simulink model "quadcopter_control"  (R2018b)
settings: Solver=VariableStepAuto  StartTime=0.0  StopTime=2.5  RelTol=1e-3
undefined symbols (not defined in the file or in its folder): armLength, dragFactor, iX, iY, iZ, mass, phi0, phiDot0, psi0, psiDot0, theta0, thetaDot0, thrustFactor, trajectory, Ts, x0, xDot0, y0, yDot0, z0, zDot0
libraries: simulink x1
settings Model: Creator=Ramprasad  LastModifiedBy=Ramprasad

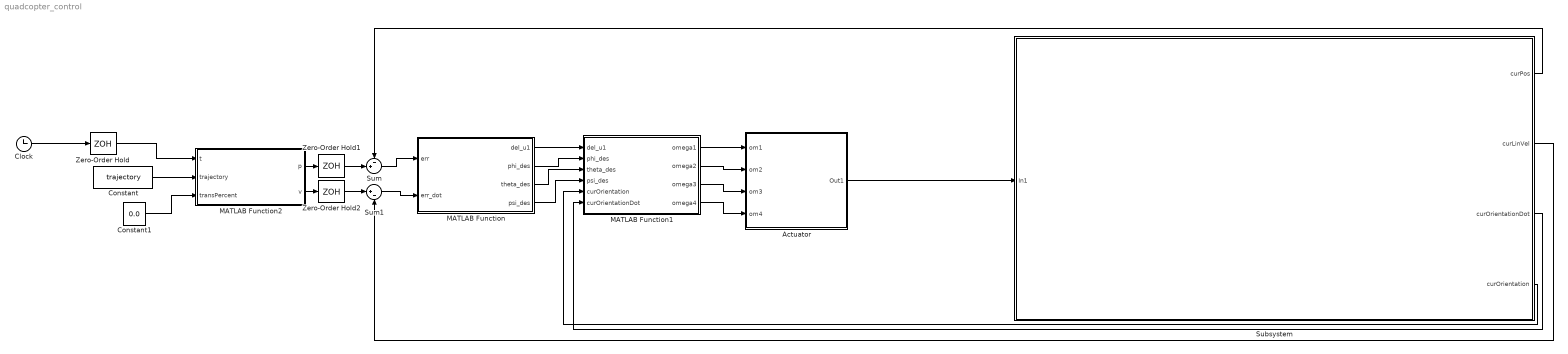
== system quadcopter_control ==
  Actuator : Subsystem
  Clock : Clock
  Constant : Constant  Value=trajectory
  Constant1 : Constant  Value=0.0
  MATLAB Function : MATLAB Function  TreatAsAtomicUnit=on
  MATLAB Function1 : MATLAB Function  TreatAsAtomicUnit=on
  MATLAB Function2 : MATLAB Function  TreatAsAtomicUnit=on
  Subsystem : Subsystem
  Sum : Sum  Inputs=-+|
  Sum1 : Sum  Inputs=|+-
  Zero-Order Hold : ZeroOrderHold  SampleTime=0.001
  Zero-Order Hold1 : ZeroOrderHold  SampleTime=0.001
  Zero-Order Hold2 : ZeroOrderHold  SampleTime=0.001
  wires:
  Actuator/1(Out1) -> Subsystem/1(In1)
  Constant/1 -> MATLAB Function2/2(trajectory)
  Clock/1 -> Zero-Order Hold/1
  Zero-Order Hold/1 -> MATLAB Function2/1(t)
  Subsystem/3(curOrientationDot) -> MATLAB Function1/6(curOrientationDot)
  Subsystem/4(curOrientation) -> MATLAB Function1/5(curOrientation)
  MATLAB Function/1(del_u1) -> MATLAB Function1/1(del_u1)
  MATLAB Function/2(phi_des) -> MATLAB Function1/2(phi_des)
  MATLAB Function/3(theta_des) -> MATLAB Function1/3(theta_des)
  MATLAB Function/4(psi_des) -> MATLAB Function1/4(psi_des)
  MATLAB Function2/1(p) -> Zero-Order Hold1/1
  MATLAB Function2/2(v) -> Zero-Order Hold2/1
  Zero-Order Hold1/1 -> Sum/2
  Zero-Order Hold2/1 -> Sum1/1
  Sum/1 -> MATLAB Function/1(err)
  Sum1/1 -> MATLAB Function/2(err_dot)
  MATLAB Function1/1(omega1) -> Actuator/1(om1)
  MATLAB Function1/2(omega2) -> Actuator/2(om2)
  MATLAB Function1/3(omega3) -> Actuator/3(om3)
  MATLAB Function1/4(omega4) -> Actuator/4(om4)
  Subsystem/2(curLinVel) -> Sum1/2
  Subsystem/1(curPos) -> Sum/1
  Constant1/1 -> MATLAB Function2/3(transPercent)

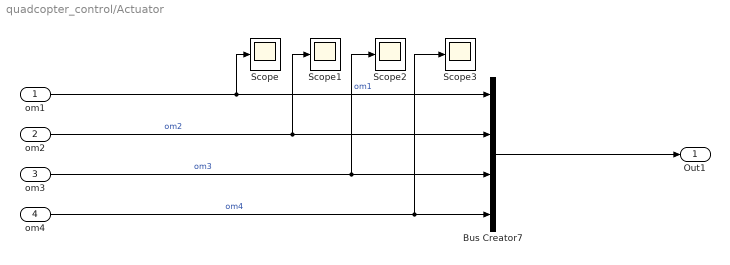
== system quadcopter_control/Actuator ==
  om1 : Inport
  om2 : Inport  Port=2
  om3 : Inport  Port=3
  om4 : Inport  Port=4
  Bus Creator7 : BusCreator  Inputs=4
  Scope{,1..3} (4 alike) : Scope
  Out1 : Outport
  wires:
  om1/1 -> Scope/1, Bus Creator7/1  "om1"
  om4/1 -> Scope3/1, Bus Creator7/4  "om4"
  Bus Creator7/1 -> Out1/1
  om2/1 -> Scope1/1, Bus Creator7/2  "om2"
  om3/1 -> Scope2/1, Bus Creator7/3  "om3"

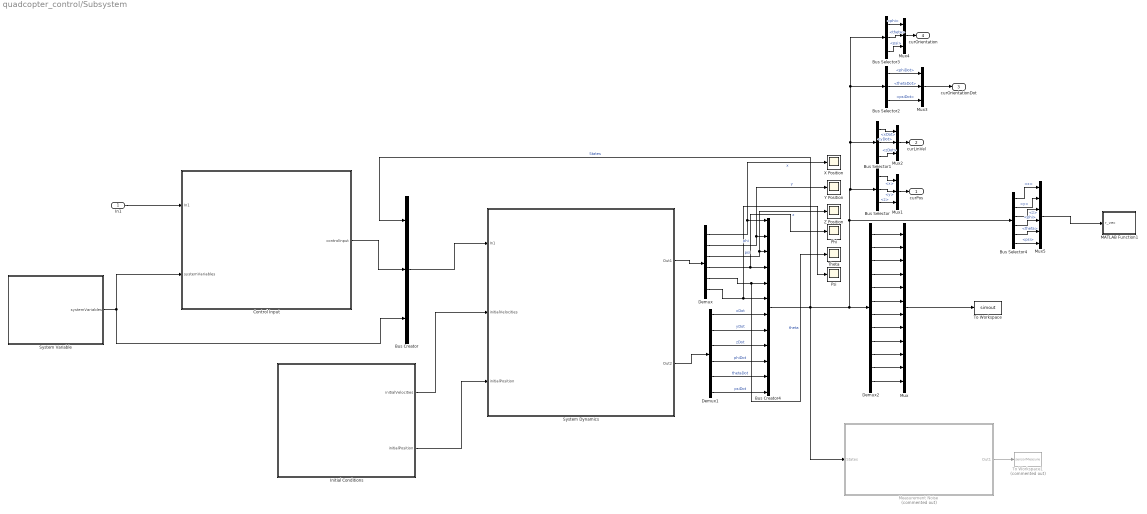
== system quadcopter_control/Subsystem ==
  In1 : Inport
  Bus Creator : BusCreator  Inputs=3
  Bus Creator4 : BusCreator  Inputs=12
  Bus Selector : BusSelector  OutputSignals=x,y,z
  Bus Selector1 : BusSelector  OutputSignals=xDot,yDot,zDot
  Bus Selector2 : BusSelector  OutputSignals=phiDot,thetaDot,psiDot
  Bus Selector3 : BusSelector  OutputSignals=phi,theta,psi
  Bus Selector4 : BusSelector  OutputSignals=x,y,z,phi,theta,psi
  Control Input : Subsystem
  Demux : Demux  Outputs=6
  Demux1 : Demux  Outputs=6
  Demux2 : Demux  Outputs=12
  Initial Conditions : Subsystem
  MATLAB Function1 : MATLAB Function  TreatAsAtomicUnit=on
  Measurement Noise : Subsystem  Commented=on
  Mux : Mux  Inputs=12
  Mux{1..4} (4 alike) : Mux  Inputs=3
  Mux5 : Mux  Inputs=6
  Phi : Scope
  Psi : Scope
  System Dynamics : Subsystem
  System Variable : Subsystem
  Theta : Scope
  To Workspace : ToWorkspace  VariableName=simout  SaveFormat=Timeseries  SampleTime=-1
  To Workspace1 : ToWorkspace  Commented=on  VariableName=sensorMeasure  SaveFormat=Timeseries  SampleTime=-1
  X Position : Scope
  Y Position : Scope
  Z Position : Scope
  curPos : Outport
  curLinVel : Outport  Port=2
  curOrientationDot : Outport  Port=3
  curOrientation : Outport  Port=4
  wires:
  Demux1/1 -> Bus Creator4/7  "xDot"
  Demux2/6 -> Mux/6
  Demux/6 -> Psi/1, Bus Creator4/6  "psi"
  Demux1/2 -> Bus Creator4/8  "yDot"
  Mux/1 -> To Workspace/1
  Demux2/9 -> Mux/9
  Demux1/6 -> Bus Creator4/12  "psiDot"
  Measurement Noise/1(Out1) -> To Workspace1/1
  Demux/4 -> Phi/1, Bus Creator4/4  "phi"
  System Dynamics/1(Out1) -> Demux/1
  Initial Conditions/1(initialVelocities) -> System Dynamics/2(initialVelocities)
  Initial Conditions/2(initialPosition) -> System Dynamics/3(initialPosition)
  Bus Creator/1 -> System Dynamics/1(In1)
  Demux/2 -> Bus Creator4/2, Y Position/1  "y"
  Demux2/5 -> Mux/5
  System Dynamics/2(Out2) -> Demux1/1
  Demux2/3 -> Mux/3
  Demux/1 -> Bus Creator4/1, X Position/1  "x"
  Demux2/8 -> Mux/8
  Demux2/7 -> Mux/7
  Control Input/1(controlInput) -> Bus Creator/2
  Demux2/2 -> Mux/2
  In1/1 -> Control Input/1(In1)
  Demux2/12 -> Mux/12
  Demux1/4 -> Bus Creator4/10  "phiDot"
  Demux/5 -> Theta/1, Bus Creator4/5  "theta"
  Demux/3 -> Z Position/1, Bus Creator4/3  "z"
  Demux2/1 -> Mux/1
  Demux2/10 -> Mux/10
  Bus Creator4/1 -> Bus Creator/1, Bus Selector3/1, Bus Selector2/1, Bus Selector1/1, Bus Selector/1, Bus Selector4/1, Demux2/1, Measurement Noise/1(States)  "States"
  Demux2/11 -> Mux/11
  Demux1/5 -> Bus Creator4/11  "thetaDot"
  Demux2/4 -> Mux/4
  Demux1/3 -> Bus Creator4/9  "zDot"
  System Variable/1(systemVariables) -> Control Input/2(systemVariables), Bus Creator/3
  Bus Selector/3 -> Mux1/3  "<z>"
  Bus Selector/2 -> Mux1/2  "<y>"
  Bus Selector/1 -> Mux1/1  "<x>"
  Mux1/1 -> curPos/1
  Bus Selector1/2 -> Mux2/2  "<yDot>"
  Bus Selector1/3 -> Mux2/3  "<zDot>"
  Bus Selector1/1 -> Mux2/1  "<xDot>"
  Mux2/1 -> curLinVel/1
  Bus Selector3/1 -> Mux4/1  "<phi>"
  Bus Selector3/2 -> Mux4/2  "<theta>"
  Bus Selector3/3 -> Mux4/3  "<psi>"
  Mux4/1 -> curOrientation/1
  Bus Selector2/1 -> Mux3/1  "<phiDot>"
  Bus Selector2/2 -> Mux3/2  "<thetaDot>"
  Mux3/1 -> curOrientationDot/1
  Bus Selector2/3 -> Mux3/3  "<psiDot>"
  Bus Selector4/1 -> Mux5/1  "<x>"
  Bus Selector4/2 -> Mux5/2  "<y>"
  Bus Selector4/3 -> Mux5/3  "<z>"
  Bus Selector4/4 -> Mux5/4  "<phi>"
  Bus Selector4/5 -> Mux5/5  "<theta>"
  Bus Selector4/6 -> Mux5/6  "<psi>"
  Mux5/1 -> MATLAB Function1/1(r_vec)

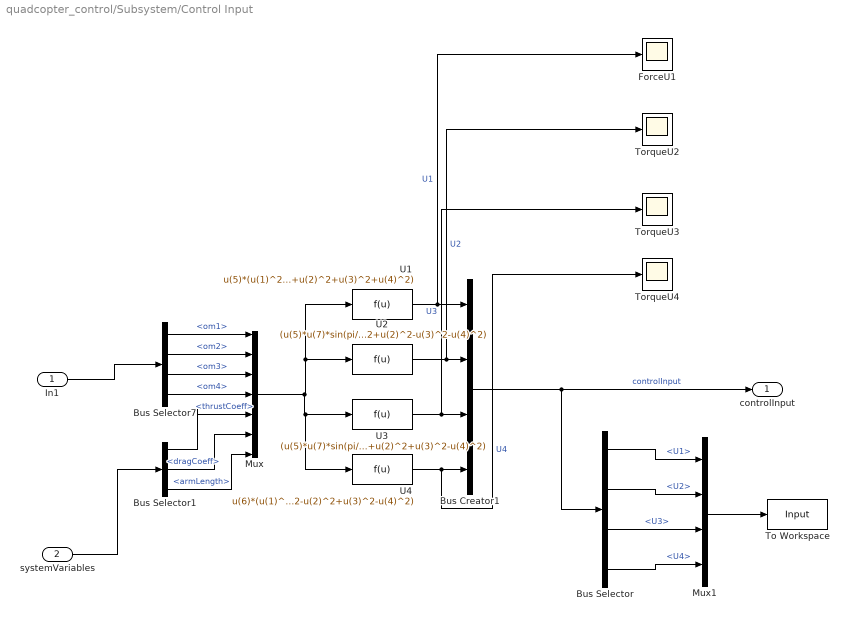
== system quadcopter_control/Subsystem/Control Input ==
  In1 : Inport
  systemVariables : Inport  Port=2
  Bus Creator1 : BusCreator  Inputs=4
  Bus Selector : BusSelector  OutputSignals=U1,U2,U3,U4
  Bus Selector1 : BusSelector  OutputSignals=thrustCoeff,dragCoeff,armLength
  Bus Selector7 : BusSelector  OutputSignals=om1,om2,om3,om4
  ForceU1 : Scope
  Mux : Mux  Inputs=7
  Mux1 : Mux
  To Workspace : ToWorkspace  VariableName=Input  SaveFormat=Timeseries  SampleTime=-1
  TorqueU2 : Scope
  TorqueU3 : Scope
  TorqueU4 : Scope
  U1 : Fcn  Expr=u(5)*(u(1)^2+u(2)^2+u(3)^2+u(4)^2)
  U2 : Fcn  Expr=(u(5)*u(7)*sin(pi/4))*(u(1)^2+u(2)^2-u(3)^2-u(4)^2)
  U3 : Fcn  Expr=(u(5)*u(7)*sin(pi/4))*(-u(1)^2+u(2)^2+u(3)^2-u(4)^2)
  U4 : Fcn  Expr=u(6)*(u(1)^2-u(2)^2+u(3)^2-u(4)^2)
  controlInput : Outport
  wires:
  Mux1/1 -> To Workspace/1
  Bus Selector/4 -> Mux1/4  "<U4>"
  Bus Selector/3 -> Mux1/3  "<U3>"
  Bus Selector/2 -> Mux1/2  "<U2>"
  Bus Selector/1 -> Mux1/1  "<U1>"
  Bus Selector7/3 -> Mux/3  "<om3>"
  In1/1 -> Bus Selector7/1
  Mux/1 -> U1/1, U2/1, U3/1, U4/1
  U1/1 -> Bus Creator1/1, ForceU1/1  "U1"
  U4/1 -> Bus Creator1/4, TorqueU4/1  "U4"
  Bus Selector1/3 -> Mux/7  "<armLength>"
  U3/1 -> Bus Creator1/3, TorqueU3/1  "U3"
  Bus Selector1/1 -> Mux/5  "<thrustCoeff>"
  Bus Creator1/1 -> controlInput/1, Bus Selector/1  "controlInput"
  Bus Selector1/2 -> Mux/6  "<dragCoeff>"
  U2/1 -> Bus Creator1/2, TorqueU2/1  "U2"
  Bus Selector7/1 -> Mux/1  "<om1>"
  Bus Selector7/4 -> Mux/4  "<om4>"
  Bus Selector7/2 -> Mux/2  "<om2>"
  systemVariables/1 -> Bus Selector1/1

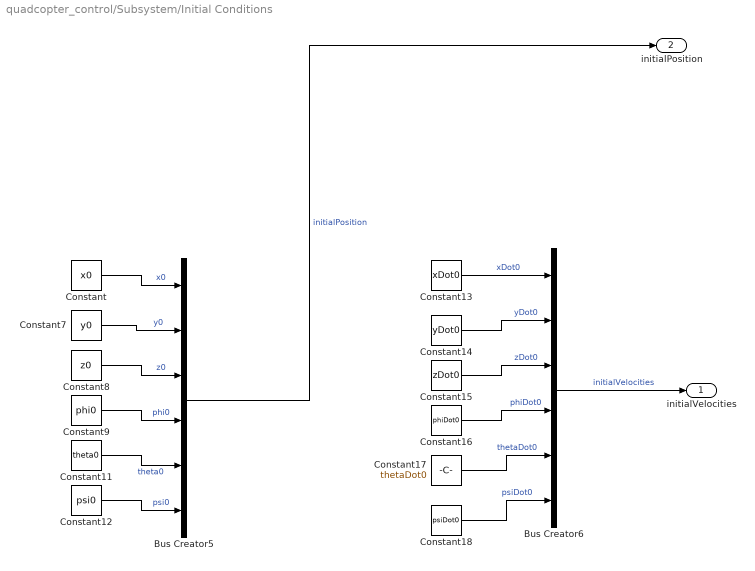
== system quadcopter_control/Subsystem/Initial Conditions ==
  Bus Creator5 : BusCreator  Inputs=6
  Bus Creator6 : BusCreator  Inputs=6
  Constant : Constant  Value=x0
  Constant11 : Constant  Value=theta0
  Constant12 : Constant  Value=psi0
  Constant13 : Constant  Value=xDot0
  Constant14 : Constant  Value=yDot0
  Constant15 : Constant  Value=zDot0
  Constant16 : Constant  Value=phiDot0
  Constant17 : Constant  Value=thetaDot0
  Constant18 : Constant  Value=psiDot0
  Constant7 : Constant  Value=y0
  Constant8 : Constant  Value=z0
  Constant9 : Constant  Value=phi0
  initialVelocities : Outport
  initialPosition : Outport  Port=2
  wires:
  Constant9/1 -> Bus Creator5/4  "phi0"
  Constant14/1 -> Bus Creator6/2  "yDot0"
  Constant17/1 -> Bus Creator6/5  "thetaDot0"
  Constant18/1 -> Bus Creator6/6  "psiDot0"
  Constant13/1 -> Bus Creator6/1  "xDot0"
  Constant11/1 -> Bus Creator5/5  "theta0"
  Constant8/1 -> Bus Creator5/3  "z0"
  Constant16/1 -> Bus Creator6/4  "phiDot0"
  Constant12/1 -> Bus Creator5/6  "psi0"
  Constant15/1 -> Bus Creator6/3  "zDot0"
  Constant/1 -> Bus Creator5/1  "x0"
  Bus Creator6/1 -> initialVelocities/1  "initialVelocities"
  Constant7/1 -> Bus Creator5/2  "y0"
  Bus Creator5/1 -> initialPosition/1  "initialPosition"

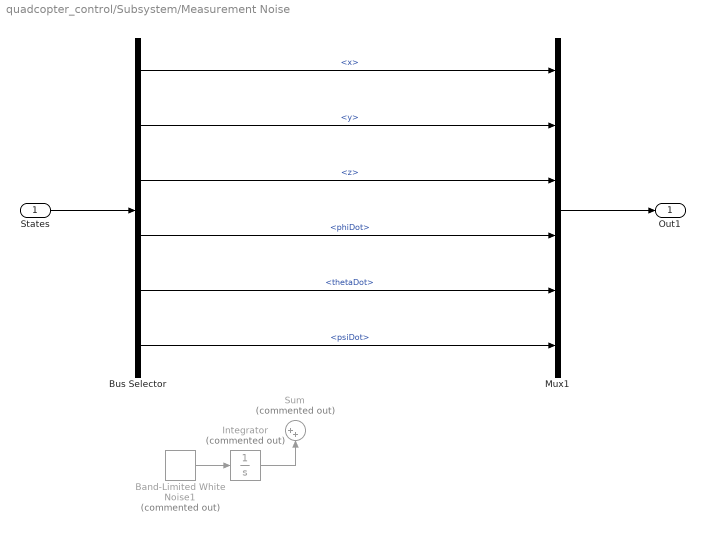
== system quadcopter_control/Subsystem/Measurement Noise ==
  States : Inport
  Band-Limited White Noise1 : simulink/Sources/Band-Limited White Noise  Commented=on  Cov=[0.0]  Ts=Ts  seed=[23341]
  Bus Selector : BusSelector  OutputSignals=x,y,z,phiDot,thetaDot,psiDot
  Integrator : Integrator  Commented=on
  Mux1 : Mux  Inputs=6
  Sum : Sum  Commented=on  Inputs=|++
  Out1 : Outport
  wires:
  Integrator/1 -> Sum/2
  Bus Selector/3 -> Mux1/3  "<z>"
  Bus Selector/2 -> Mux1/2  "<y>"
  Mux1/1 -> Out1/1
  Band-Limited White Noise1/1 -> Integrator/1
  Bus Selector/4 -> Mux1/4  "<phiDot>"
  States/1 -> Bus Selector/1
  Bus Selector/6 -> Mux1/6  "<psiDot>"
  Bus Selector/5 -> Mux1/5  "<thetaDot>"
  Bus Selector/1 -> Mux1/1  "<x>"

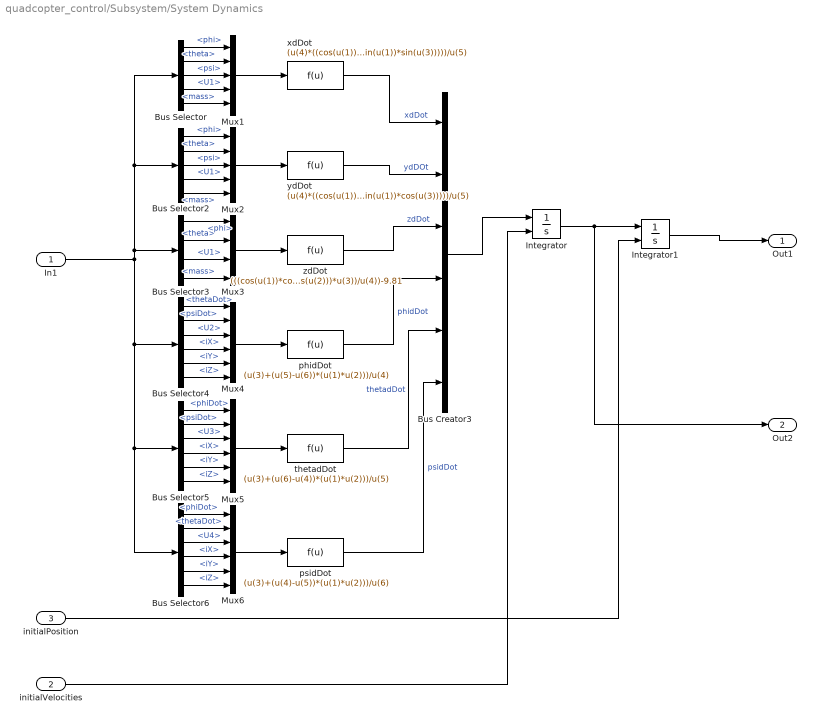
== system quadcopter_control/Subsystem/System Dynamics ==
  In1 : Inport
  initialVelocities : Inport  Port=2
  initialPosition : Inport  Port=3
  Bus Creator3 : BusCreator  Inputs=6
  Bus Selector : BusSelector  OutputSignals=States.phi,States.theta,States.psi,controlInput.U1,systemVariables.mass
  Bus Selector2 : BusSelector  OutputSignals=States.phi,States.theta,States.psi,controlInput.U1,systemVariables.mass
  Bus Selector3 : BusSelector  OutputSignals=States.phi,States.theta,controlInput.U1,systemVariables.mass
  Bus Selector4 : BusSelector  OutputSignals=States.thetaDot,States.psiDot,controlInput.U2,systemVariables.iX,systemVariables.iY,systemVariables.iZ
  Bus Selector5 : BusSelector  OutputSignals=States.phiDot,States.psiDot,controlInput.U3,systemVariables.iX,systemVariables.iY,systemVariables.iZ
  Bus Selector6 : BusSelector  OutputSignals=States.phiDot,States.thetaDot,controlInput.U4,systemVariables.iX,systemVariables.iY,systemVariables.iZ
  Integrator : Integrator  InitialConditionSource=external
  Integrator1 : Integrator  InitialConditionSource=external
  Mux1 : Mux  Inputs=5
  Mux2 : Mux  Inputs=5
  Mux3 : Mux
  Mux4 : Mux  Inputs=6
  Mux5 : Mux  Inputs=6
  Mux6 : Mux  Inputs=6
  phidDot : Fcn  Expr=(u(3)+(u(5)-u(6))*(u(1)*u(2)))/u(4)
  psidDot : Fcn  Expr=(u(3)+(u(4)-u(5))*(u(1)*u(2)))/u(6)
  thetadDot : Fcn  Expr=(u(3)+(u(6)-u(4))*(u(1)*u(2)))/u(5)
  xdDot : Fcn  Expr=(u(4)*((cos(u(1))*sin(u(2))*cos(u(3)))+(sin(u(1))*sin(u(3)))))/u(5)
  ydDot : Fcn  Expr=(u(4)*((cos(u(1))*sin(u(2))*sin(u(3)))-(sin(u(1))*cos(u(3)))))/u(5)
  zdDot : Fcn  Expr=(((cos(u(1))*cos(u(2)))*u(3))/u(4))-9.81
  Out1 : Outport
  Out2 : Outport  Port=2
  wires:
  initialPosition/1 -> Integrator1/2
  xdDot/1 -> Bus Creator3/1  "xdDot"
  Bus Selector2/2 -> Mux2/2  "<theta>"
  Bus Selector4/5 -> Mux4/5  "<iY>"
  Bus Selector2/4 -> Mux2/4  "<U1>"
  Bus Selector4/3 -> Mux4/3  "<U2>"
  thetadDot/1 -> Bus Creator3/5  "thetadDot"
  Bus Selector5/2 -> Mux5/2  "<psiDot>"
  Bus Selector2/1 -> Mux2/1  "<phi>"
  Mux5/1 -> thetadDot/1
  Bus Selector6/4 -> Mux6/4  "<iX>"
  Bus Selector5/6 -> Mux5/6  "<iZ>"
  Bus Selector6/2 -> Mux6/2  "<thetaDot>"
  phidDot/1 -> Bus Creator3/4  "phidDot"
  Bus Selector2/3 -> Mux2/3  "<psi>"
  In1/1 -> Bus Selector4/1, Bus Selector5/1, Bus Selector6/1, Bus Selector3/1, Bus Selector2/1, Bus Selector/1
  Bus Selector5/3 -> Mux5/3  "<U3>"
  Bus Selector3/2 -> Mux3/2  "<theta>"
  Bus Selector3/1 -> Mux3/1  "<phi>"
  initialVelocities/1 -> Integrator/2
  Bus Selector/3 -> Mux1/3  "<psi>"
  Mux6/1 -> psidDot/1
  Bus Selector5/4 -> Mux5/4  "<iX>"
  Bus Selector/4 -> Mux1/4  "<U1>"
  Bus Selector/1 -> Mux1/1  "<phi>"
  Mux4/1 -> phidDot/1
  Bus Selector4/6 -> Mux4/6  "<iZ>"
  Bus Selector2/5 -> Mux2/5  "<mass>"
  Bus Creator3/1 -> Integrator/1
  Bus Selector6/6 -> Mux6/6  "<iZ>"
  Bus Selector3/3 -> Mux3/3  "<U1>"
  Mux2/1 -> ydDot/1
  Bus Selector6/3 -> Mux6/3  "<U4>"
  Bus Selector6/1 -> Mux6/1  "<phiDot>"
  zdDot/1 -> Bus Creator3/3  "zdDot"
  Bus Selector5/1 -> Mux5/1  "<phiDot>"
  Bus Selector4/2 -> Mux4/2  "<psiDot>"
  Bus Selector6/5 -> Mux6/5  "<iY>"
  Bus Selector4/4 -> Mux4/4  "<iX>"
  Bus Selector4/1 -> Mux4/1  "<thetaDot>"
  Mux3/1 -> zdDot/1
  Integrator/1 -> Integrator1/1, Out2/1
  psidDot/1 -> Bus Creator3/6  "psidDot"
  Integrator1/1 -> Out1/1
  Bus Selector/5 -> Mux1/5  "<mass>"
  ydDot/1 -> Bus Creator3/2  "ydDOt"
  Bus Selector5/5 -> Mux5/5  "<iY>"
  Bus Selector/2 -> Mux1/2  "<theta>"
  Bus Selector3/4 -> Mux3/4  "<mass>"
  Mux1/1 -> xdDot/1

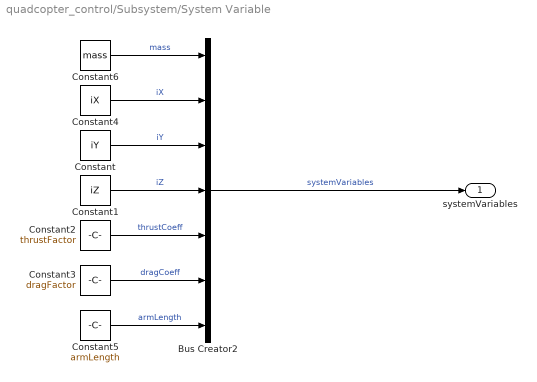
== system quadcopter_control/Subsystem/System Variable ==
  Bus Creator2 : BusCreator  Inputs=7
  Constant : Constant  Value=iY
  Constant1 : Constant  Value=iZ
  Constant2 : Constant  Value=thrustFactor
  Constant3 : Constant  Value=dragFactor
  Constant4 : Constant  Value=iX
  Constant5 : Constant  Value=armLength
  Constant6 : Constant  Value=mass
  systemVariables : Outport
  wires:
  Constant6/1 -> Bus Creator2/1  "mass"
  Constant2/1 -> Bus Creator2/5  "thrustCoeff"
  Constant/1 -> Bus Creator2/3  "iY"
  Constant1/1 -> Bus Creator2/4  "iZ"
  Constant3/1 -> Bus Creator2/6  "dragCoeff"
  Constant4/1 -> Bus Creator2/2  "iX"
  Constant5/1 -> Bus Creator2/7  "armLength"
  Bus Creator2/1 -> systemVariables/1  "systemVariables"

== matlab function quadcopter_control/Subsystem/MATLAB Function1 ==
  settings: updateMethod=DISCRETE
  data: r_vec input
function drawDrone(r_vec)
%#codegen
coder.extrinsic('evalin');
coder.extrinsic('load');
% persistent figNum axisHandel Sim_Exact points3D;

% if isempty(Sim_Exact)
%     Sim_Exact = evalin('base','Sim_Exact');
%     a.points3D = zeros(21,3,'double');
%     a = load('points3D.mat');
%     points3D = zeros(21,3,'double');
%     points3D = a.points3D;
% end

x = r_vec(1);
y = r_vec(2);
z = r_vec(3);
phi = r_vec(4);
theta = r_vec(5);
psi = r_vec(6);

T06 = [cos(psi)*cos(theta) (cos(psi)*sin(theta)*sin(phi))-(sin(psi)*cos(phi)) (cos(phi)*sin(theta)*cos(psi))+(sin(phi)*sin(psi)) x;...
       sin(psi)*cos(theta) (sin(phi)*sin(theta)*sin(psi))+(cos(phi)*cos(psi)) (sin(psi)*sin(theta)*cos(phi))-(cos(psi)*sin(phi)) y;...
       -sin(theta) (cos(theta)*sin(phi)) (cos(theta)*cos(phi)) z;...
       0 0 0 1];

R06 = T06(1:3,1:3);

% P1 =[ 0
%     0
%     0.29];
% P2 = [ 0.27*cos(x)*cos(y);
%     0.27*cos(y)*sin(x);
%     0.29 - 0.27*sin(y)];
% P3 = [ 0.27*cos(x)*cos(y) - 0.07*cos(x)*sin(y)*sin(z) + 0.07*cos(x)*cos(y)*cos(z);
%     0.27*cos(y)*sin(x) - 0.07*sin(x)*sin(y)*sin(z) + 0.07*cos(y)*cos(z)*sin(x);
%     0.29 - 0.07*cos(y)*sin(z) - 0.07*cos(z)*sin(y) - 0.27*sin(y)];
% 
% P4 = [ 0.27*cos(x)*cos(y) - 0.07*cos(x)*sin(y)*sin(z) + 0.07*cos(x)*cos(y)*cos(z) - 0.302*cos(x)*cos(y)*sin(z) - 0.302*cos(x)*cos(z)*sin(y);
%     0.27*cos(y)*sin(x) - 0.302*cos(y)*sin(x)*sin(z) - 0.302*cos(z)*sin(x)*sin(y) - 0.07*sin(x)*sin(y)*sin(z) + 0.07*cos(y)*cos(z)*sin(x);
%     0.302*sin(y)*sin(z) - 0.302*cos(y)*cos(z) - 0.07*cos(y)*sin(z) - 0.07*cos(z)*sin(y) - 0.27*sin(y) + 0.29];
% P5 = [ 0.27*cos(x)*cos(y) - 0.07*cos(x)*sin(y)*sin(z) + 0.07*cos(x)*cos(y)*cos(z) - 0.302*cos(x)*cos(y)*sin(z) - 0.302*cos(x)*cos(z)*sin(y)
%     0.27*cos(y)*sin(x) - 0.302*cos(y)*sin(x)*sin(z) - 0.302*cos(z)*sin(x)*sin(y) - 0.07*sin(x)*sin(y)*sin(z) + 0.07*cos(y)*cos(z)*sin(x)
%     0.302*sin(y)*sin(z) - 0.302*cos(y)*cos(z) - 0.07*cos(y)*sin(z) - 0.07*cos(z)*sin(y) - 0.27*sin(y) + 0.29];
% 
% P6 =[ 0.27*cos(x)*cos(y) - 0.07*cos(x)*sin(y)*sin(z) - 0.072*sin(x)*sin(phi)*sin(theta) + 0.07*cos(x)*cos(y)*cos(z) - 0.302*cos(x)*cos(y)*sin(z) - 0.302*cos(x)*cos(z)*sin(y) - 0.072*cos(x)*cos(y)*cos(theta)*sin(z) - 0.072*cos(x)*cos(z)*cos(theta)*sin(y) - 0.072*cos(x)*cos(y)*cos(z)*cos(phi)*sin(theta) + 0.072*cos(x)*cos(phi)*sin(y)*sin(z)*sin(theta);
%     0.27*cos(y)*sin(x) - 0.302*cos(y)*sin(x)*sin(z) - 0.302*cos(z)*sin(x)*sin(y) + 0.072*cos(x)*sin(phi)*sin(theta) - 0.07*sin(x)*sin(y)*sin(z) + 0.07*cos(y)*cos(z)*sin(x) - 0.072*cos(y)*cos(theta)*sin(x)*sin(z) - 0.072*cos(z)*cos(theta)*sin(x)*sin(y) - 0.072*cos(y)*cos(z)*cos(phi)*sin(x)*sin(theta) + 0.072*cos(phi)*sin(x)*sin(y)*sin(z)*sin(theta);
%     0.302*sin(y)*sin(z) - 0.302*cos(y)*cos(z) - 0.07*cos(y)*sin(z) - 0.07*cos(z)*sin(y) - 0.27*sin(y) + 0.072*cos(theta)*sin(y)*sin(z) - 0.072*cos(y)*cos(z)*cos(theta) + 0.072*cos(y)*cos(phi)*sin(z)*sin(theta) + 0.072*cos(z)*cos(phi)*sin(y)*sin(theta) + 0.29];

Q1 = [(0.1/sqrt(2));(0.1/sqrt(2));0];
Q2 = [-(0.1/sqrt(2));(0.1/sqrt(2));0];
Q3 = [(0.1/sqrt(2));-(0.1/sqrt(2));0];
Q4 = [-(0.1/sqrt(2));-(0.1/sqrt(2));0];

R1 = R06*Q1;
R2 = R06*Q2;
R3 = R06*Q3;
R4 = R06*Q4;

P1 = [x+R1(1);y+R1(2);z+R1(3)];
P2 = [x+R2(1);y+R2(2);z+R2(3)];
P3 = [x+R3(1);y+R3(2);z+R3(3)];
P4 = [x+R4(1);y+R4(2);z+R4(3)];

% if isempty(figNum)
%     figNum = figure(1);
%     hold on;
%     plot3([0;P1(1);P2(1);P3(1);P4(1);P5(1);P6(1)],...
%         [0;P1(2);P2(2);P3(2);P4(2);P5(2);P6(2)],...
%         [0;P1(3);P2(3);P3(3);P4(3);P5(3);P6(3)],'k','linewidth',2);
%     axisHandel = gca;
%     plot3([P6(1);P6(1)+T06(1,1)*.1],...
%         [P6(2);P6(2)+T06(2,1)*.1],...
%         [P6(3);P6(3)+T06(3,1)*.1],'r','Parent',axisHandel);
%     plot3([P6(1);P6(1)+T06(1,2)*.1],...
%         [P6(2);P6(2)+T06(2,2)*.1],...
%         [P6(3);P6(3)+T06(3,2)*.1],'g','Parent',axisHandel);
%     plot3([P6(1);P6(1)+T06(1,3)*.1],...
%         [P6(2);P6(2)+T06(2,3)*.1],...
%         [P6(3);P6(3)+T06(3,3)*.1],'b','Parent',axisHandel);
%     plot3(points3D(:,1),points3D(:,2),points3D(:,3),'m','Parent',axisHandel);
%     hold off;
%     axis([-.75 .75 -.75 .75 -.4 .75]);
%     axisHandel = gca;
% else
plot3([x;P1(1)],[y;P1(2)],[z;P1(3)],'k','linewidth',2,'Parent',gca);
hold on;
plot3([x;P2(1)],[y;P2(2)],[z;P2(3)],'k','linewidth',2,'Parent',gca);
hold on;
plot3([x;P3(1)],[y;P3(2)],[z;P3(3)],'k','linewidth',2,'Parent',gca);
hold on;
plot3([x;P4(1)],[y;P4(2)],[z;P4(3)],'k','linewidth',2,'Parent',gca);
hold on;
plot3([x;x+T06(1,1)*.1],[y;y+T06(2,1)*.1],[z;z+T06(3,1)*.1],'r','Parent',gca);
plot3([x;x+T06(1,2)*.1],[y;y+T06(2,2)*.1],[z;z+T06(3,2)*.1],'g','Parent',gca);
plot3([x;x+T06(1,3)*.1],[y;y+T06(2,3)*.1],[z;z+T06(3,3)*.1],'b','Parent',gca);
% plot3([P6(1);P6(1)+T06(1,2)*.1],...
%     [P6(2);P6(2)+T06(2,2)*.1],...
%     [P6(3);P6(3)+T06(3,2)*.1],'g','Parent',gca);
% plot3([P6(1);P6(1)+T06(1,3)*.1],...
%     [P6(2);P6(2)+T06(2,3)*.1],...
%     [P6(3);P6(3)+T06(3,3)*.1],'b','Parent',gca);
% plot3(points3D(:,1),points3D(:,2),points3D(:,3),'m','Parent',gca);
hold off;
%axis([-.75 .75 -.75 .75 -.4 .75]*10);
end

== matlab function quadcopter_control/MATLAB Function2 ==
  data: t input; p output; trajectory input; transPercent input; v output
function [p,v] = constAccelInterp(t,trajectory,transPercent)
pTime = trajectory(:,1);
[n,m] = size(trajectory);
p = zeros(1,m-1);
v = zeros(1,m-1);
a = zeros(1,m-1);
for j = 2:n-1
    if j-1==1 && t>pTime(j-1,1) && t<(pTime(j-1,1)+transPercent)
        for i = 2:m
            p(1,i-1) = trajectory(j-1,i) +...
                (((trajectory(j,i)-trajectory(j-1,i))*((t-pTime(j-1,1)+transPercent)^2))/(4*transPercent*(pTime(j,1)-pTime(j-1,1))));
            v(1,i-1) = (((trajectory(j,i)-trajectory(j-1,i))*(t-pTime(j-1,1)+transPercent))/(2*transPercent*(pTime(j,1)-pTime(j-1,1))));
            a(1,i-1) = ((trajectory(j,i)-trajectory(j-1,i))/(2*transPercent*(pTime(j,1)-pTime(j-1,1))));
        end
        break;
    elseif j+1==n && t>(pTime(j+1,1)-transPercent) && t<pTime(j+1,1)
        for i = 2:m
            p(1,i-1) = trajectory(j+1,i) - ...
                (((trajectory(j+1,i)-trajectory(j,i))*((t-pTime(j+1,1)-transPercent)^2))/(4*transPercent*(pTime(j+1,1)-pTime(j,1))));
            v(1,i-1) = -(((trajectory(j+1,i)-trajectory(j,i))*(t-pTime(j+1,1)-transPercent))/(2*transPercent*(pTime(j+1,1)-pTime(j,1))));
            a(1,i-1) = -((trajectory(j+1,i)-trajectory(j,i))/(2*transPercent*(pTime(j+1,1)-pTime(j,1))));
        end
        break;
    elseif t>(pTime(j-1,1)+transPercent) && t<(pTime(j,1)-transPercent)
        for i = 2:m
            p(1,i-1) = trajectory(j,i)-(((pTime(j,1)-t)*(trajectory(j,i)-...
                trajectory(j-1,i)))/(pTime(j,1)-pTime(j-1,1)));
            v(1,i-1) = (trajectory(j,i)-trajectory(j-1,i))/(pTime(j,1)-pTime(j-1,1));
            a(1,i-1) = 0.0;
        end
        break;
    elseif t>(pTime(j,1)-transPercent) && t<(pTime(j,1)+transPercent)
        for i = 2:m
            p(1,i-1) = trajectory(j,i) - ...
                (((trajectory(j,i)-trajectory(j-1,i))*((t-pTime(j,1)-transPercent)^2))/(4*transPercent*(pTime(j,1)-pTime(j-1,1)))) +...
                (((trajectory(j+1,i)-trajectory(j,i))*((t-pTime(j,1)+transPercent)^2))/(4*transPercent*(pTime(j+1,1)-pTime(j,1))));
            v(1,i-1) = -(((trajectory(j,i)-trajectory(j-1,i))*(t-pTime(j,1)-transPercent))/(2*transPercent*(pTime(j,1)-pTime(j-1,1)))) +...
                (((trajectory(j+1,i)-trajectory(j,i))*(t-pTime(j,1)+transPercent))/(2*transPercent*(pTime(j+1,1)-pTime(j,1))));
            a(1,i-1) = -((trajectory(j,i)-trajectory(j-1,i))/(2*transPercent*(pTime(j,1)-pTime(j-1,1)))) + ...
                ((trajectory(j+1,i)-trajectory(j,i))/(2*transPercent*(pTime(j+1,1)-pTime(j,1))));
        end
        break;
    elseif t>(pTime(j,1)+transPercent) && t<(pTime(j+1,1)-transPercent)
        for i = 2:m
            p(1,i-1) = trajectory(j,i)+(((t-pTime(j,1))*(trajectory(j+1,i)-...
                trajectory(j,i)))/(pTime(j+1,1)-pTime(j,1)));
            v(1,i-1) = (trajectory(j+1,i)-trajectory(j,i))/(pTime(j+1,1)-pTime(j,1));
            a(1,i-1) = 0.0;
        end
        break;
    end
end
end

== matlab function quadcopter_control/MATLAB Function ==
  data: err input; err_dot input; del_u1 output; phi_des output; theta_des output; psi_des output
function [del_u1,phi_des,theta_des,psi_des] = POS_contol(err, err_dot)
%
kP = 20.0;
kD = 0.0;
psiDes = 0.0;
%
delOmegaH = sqrt((0.25*9.81)/(4*0.1));
%
r_ddot = kP*err + kD*err_dot;
%
rx_ddot = r_ddot(1);
ry_ddot = r_ddot(2);
rz_ddot = r_ddot(3);
%
del_u1 = 0.25*rz_ddot/(8*0.1*delOmegaH);
psi_des = psiDes;
%phi_des = ((rx_ddot*tan(psiDes) - ry_ddot)/rz_ddot)/(tan(psiDes)*sin(psiDes)+cos(psiDes));
%theta_des = ((rx_ddot/rz_ddot) - phi_des*sin(psiDes))/cos(psiDes);
phi_des = (rx_ddot*sin(psiDes) - ry_ddot*cos(psiDes))/9.81;
theta_des = (rx_ddot*cos(psiDes) + ry_ddot*sin(psiDes))/9.81;
%
end

== matlab function quadcopter_control/MATLAB Function1 ==
  data: del_u1 input; phi_des input; theta_des input; psi_des input; curOrientation input; omega1 output; curOrientationDot input; omega2 output; omega3 output; omega4 output
function [omega1, omega2, omega3, omega4] = Attitude_contol(del_u1,phi_des,theta_des,psi_des,curOrientation,curOrientationDot)
%
kP_Att = 1.0;
kD_Att = 0.0;
%
err = [phi_des;theta_des;psi_des] - curOrientation;
errDot = -1*curOrientationDot;
%
delOmega = kP_Att*err + kD_Att*errDot;
%
delPhi = delOmega(1);
delTheta = delOmega(2);
delPsi = delOmega(3);
%
delOmegaH = sqrt((0.25*9.81)/(4*0.1));
%
delOmegaVec = [delOmegaH + del_u1;delPhi;delTheta;delPsi];
%
R = [1 1 -1 1;1 1 1 -1;1 -1 1 1;1 -1 -1 -1];
%
omega1 = R(1,:)*delOmegaVec;
omega2 = R(2,:)*delOmegaVec;
omega3 = R(3,:)*delOmegaVec;
omega4 = R(4,:)*delOmegaVec;
%
end
